simulink model "FirstDeb"  (R2022a)
settings: Solver=VariableStepAuto  StartTime=0.0  StopTime=Time*20000  RelTol=1e-3
InitFcn:
  | Time = 40;
values from neighbouring files (symbols this model uses):
  alpha = 0.4    [First.m]
  Fixeda = fi(a,1,13,12)    [First.m]
  FixedR = fi(R,1,8,6)    [First.m]
libraries: sim_stud_lib_r2022a x5, dspsrcs4 x2, dspsigops x2
settings Model: Creator=RolePups  LastModifiedBy=RolePups

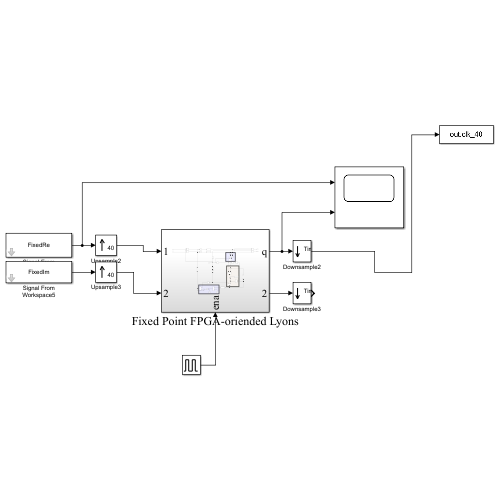
[thumbnail: Simulink's stored preview of the top-level diagram]
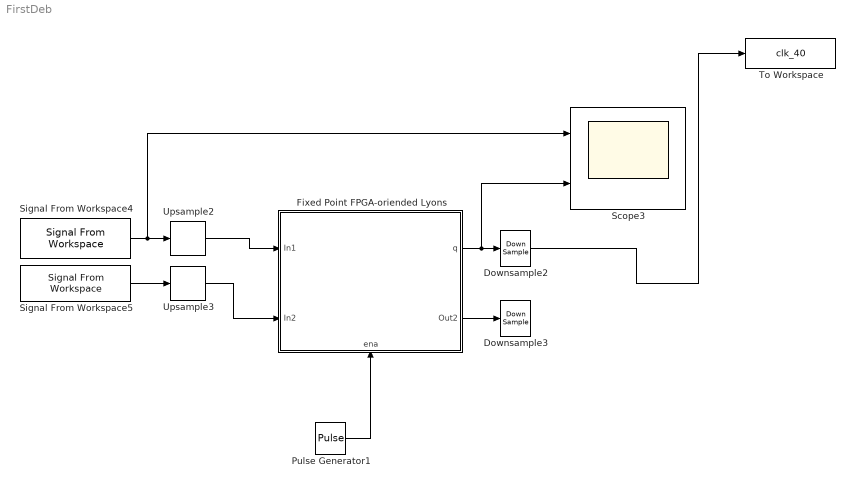
== system FirstDeb ==
  Downsample2 : DownSample  N=Time  RateOptions=Allow multirate processing
  Downsample3 : DownSample  N=Time  RateOptions=Allow multirate processing
  Fixed Point FPGA-oriended Lyons : Subsystem
      settings: PortSchema="{\"entries\":[{\"content\":{\"sides\":[{\"content\":{\"connectorIds\":[\"In1\",\"In2\"]},\"type\":\"ConnectorPlacement.EquallySpacedRectSide\",\"uuid\":\"2382ef4f-8b23-4fd9-9999-ae4ff3838c30\"},{\"content\":{\"connectorIds\":[\"Out1\",\"Out2\"],\"side\":\"RIGHT\"},\"type\":\"ConnectorPlacement.EquallySpacedRectSide\",\"uuid\":\"ff744322-ad90-46d9-948c-0637f52c7b9c\"},{\"content\":{\"connectorIds\":[],\"side\":\"TOP\"},\"type\":\"ConnectorPlacement.EquallySpacedRectSide\",\"uuid\":\"b0276f26-9e78-4e39-abf6-7a1348b88309\"},{\"content\":{\"connectorIds\":[\"In3\"],\"side\":\"BOTTOM\"},\"type\":\"ConnectorPlacement.EquallySpacedRectSide\",\"uuid\":\"b0dd70ff-8907-4b14-a46e-e3bbf4bdcae4\"}]},\"type\":\"ConnectorPlacement.EquallySpacedConnector\",\"uuid\":\"3f5cde89-4d4f-4bf7-b554-70cc79020603\"}],\"packageUris\":[\"http://schema.mathworks.com/mf0/Connector/R2020b\"],\"version\":\"1.0\"}"
  Pulse Generator1 : DiscretePulseGenerator  PulseType=Time based  Period=Time  PulseWidth=1/Time*100
  Scope3 : Scope  NumInputPorts=2
  Signal From Workspace4 : dspsrcs4/Signal From Workspace  X=FixedRe  Ts=Time  nsamps=1  OutputAfterFinalValue=Setting to zero  ignoreOrWarnInputAndFrameLengths=off  OutputFrames=off
  Signal From Workspace5 : dspsrcs4/Signal From Workspace  X=FixedIm  Ts=Time  nsamps=1  OutputAfterFinalValue=Setting to zero  ignoreOrWarnInputAndFrameLengths=off  OutputFrames=off
  To Workspace : ToWorkspace  VariableName=clk_40  SampleTime=-1
  Upsample2 : dspsigops/Upsample  N=Time  phase=0  RateOptions=Allow multirate processing  ic=0  mode=Unused parameter value
  Upsample3 : dspsigops/Upsample  N=Time  phase=0  RateOptions=Allow multirate processing  ic=0  mode=Unused parameter value
  wires:
  Fixed Point FPGA-oriended Lyons/1(q) -> Scope3/2, Downsample2/1
  Signal From Workspace5/1 -> Upsample3/1
  Upsample2/1 -> Fixed Point FPGA-oriended Lyons/1(In1)
  Fixed Point FPGA-oriended Lyons/2(Out2) -> Downsample3/1
  Pulse Generator1/1 -> Fixed Point FPGA-oriended Lyons/3(ena)
  Downsample2/1 -> To Workspace/1
  Signal From Workspace4/1 -> Scope3/1, Upsample2/1
  Upsample3/1 -> Fixed Point FPGA-oriended Lyons/2(In2)

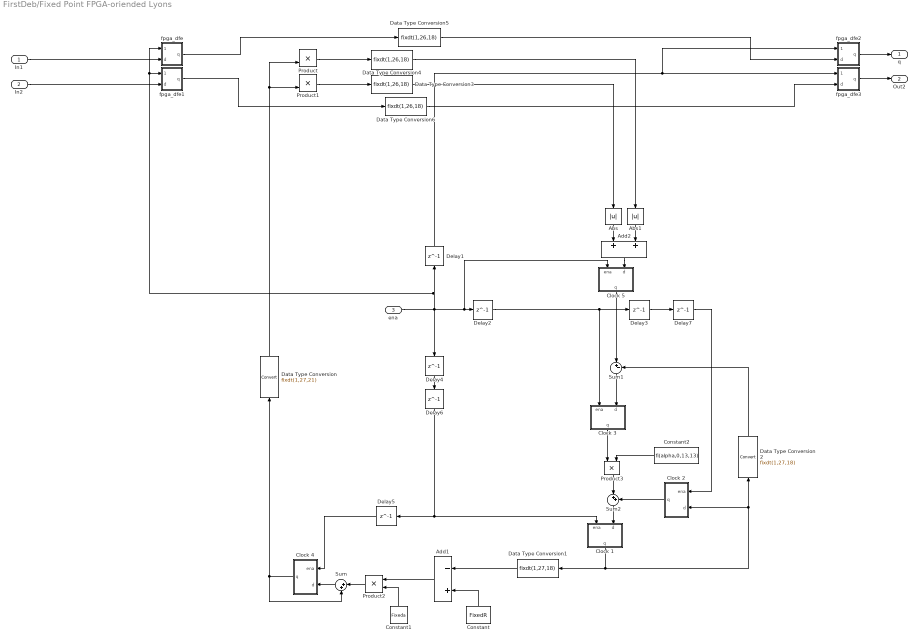
== system FirstDeb/Fixed Point FPGA-oriended Lyons ==
  In1 : Inport
  In2 : Inport  Port=2
  ena : Inport  Port=3
  Abs : Abs  OutDataTypeStr=fixdt(0,26,18)  SaturateOnIntegerOverflow=off
  Abs1 : Abs  OutDataTypeStr=fixdt(0,26,18)  SaturateOnIntegerOverflow=off
  Add1 : Sum  Inputs=-+  AccumDataTypeStr=fixdt(1,27,18)  OutDataTypeStr=fixdt(1,27,18)
  Add2 : Sum  AccumDataTypeStr=fixdt(0,27,18)  OutDataTypeStr=fixdt(0,27,18)
  Clock 1 : Subsystem
  Clock 2 : Subsystem
  Clock 3 : Subsystem
  Clock 4 : Subsystem
  Clock 5 : Subsystem
  Constant : Constant  Value=FixedR  SampleTime=-1
  Constant1 : Constant  Value=Fixeda  SampleTime=-1
  Constant2 : Constant  Value=fi(alpha,0,13,13)  SampleTime=-1
  Data Type Conversion : DataTypeConversion  OutDataTypeStr=fixdt(1,27,21)  SaturateOnIntegerOverflow=off  RndMeth=Floor
  Data Type Conversion1 : DataTypeConversion  OutDataTypeStr=fixdt(1,27,18)  SaturateOnIntegerOverflow=off  RndMeth=Floor
  Data Type Conversion2 : DataTypeConversion  OutDataTypeStr=fixdt(1,27,18)  SaturateOnIntegerOverflow=off  RndMeth=Floor
  Data Type Conversion{3..6} (4 alike) : DataTypeConversion  OutDataTypeStr=fixdt(1,26,18)  SaturateOnIntegerOverflow=off  RndMeth=Floor
  Delay{1..7} (7 alike) : Delay  DelayLength=1  InitialCondition=0
  Product : Product  OutDataTypeStr=fixdt(1,43,35)  LockScale=on
  Product1 : Product  OutDataTypeStr=fixdt(1,43,35)  LockScale=on
  Product2 : Product  OutDataTypeStr=fixdt(1,48,32)
  Product3 : Product  OutDataTypeStr=fixdt(1,48,32)
  Sum : Sum  Inputs=|++  AccumDataTypeStr=fixdt(1,48,32)  OutDataTypeStr=fixdt(1,48,32)
  Sum1 : Sum  Inputs=|+-  AccumDataTypeStr=fixdt(1,27,18)  OutDataTypeStr=fixdt(1,27,18)
  Sum2 : Sum  Inputs=|++  AccumDataTypeStr=fixdt(1,48,32)  OutDataTypeStr=fixdt(1,48,32)
  fpga_dfe : Subsystem  AncestorBlock=sim_stud_lib_r2022a/fpga_dfe
      mask Display:
      | disp('D');
      | port_label('input',1,'e');
      | port_label('input',2,'d');
      | port_label('output',1,'q');
  fpga_dfe1 : Subsystem  AncestorBlock=sim_stud_lib_r2022a/fpga_dfe
      mask Display:
      | disp('D');
      | port_label('input',1,'e');
      | port_label('input',2,'d');
      | port_label('output',1,'q');
  fpga_dfe2 : Subsystem  AncestorBlock=sim_stud_lib_r2022a/fpga_dfe
      mask Display:
      | disp('D');
      | port_label('input',1,'e');
      | port_label('input',2,'d');
      | port_label('output',1,'q');
  fpga_dfe3 : Subsystem  AncestorBlock=sim_stud_lib_r2022a/fpga_dfe
      mask Display:
      | disp('D');
      | port_label('input',1,'e');
      | port_label('input',2,'d');
      | port_label('output',1,'q');
  q : Outport
  Out2 : Outport  Port=2
  wires:
  Clock 4/1(q) -> Sum/2, Data Type Conversion/1
  Product/1 -> Data Type Conversion4/1
  Product1/1 -> Data Type Conversion3/1
  Constant/1 -> Add1/2
  Sum/1 -> Clock 4/2(d)
  Product2/1 -> Sum/1
  Constant1/1 -> Product2/2
  Abs1/1 -> Add2/2
  Abs/1 -> Add2/1
  Sum1/1 -> Clock 3/2(d)
  Constant2/1 -> Product3/2
  Product3/1 -> Sum2/1
  Clock 2/1(q) -> Sum2/2
  Add1/1 -> Product2/1
  Sum2/1 -> Clock 1/2(d)
  Clock 1/1(q) -> Data Type Conversion2/1, Clock 2/2(d), Data Type Conversion1/1
  Clock 3/1(q) -> Product3/1
  fpga_dfe2/1(q) -> q/1
  fpga_dfe3/1(q) -> Out2/1
  ena/1 -> Delay4/1, Delay1/1, fpga_dfe1/1(ena), fpga_dfe/1(ena), Clock 5/1(ena), Delay2/1
  Delay2/1 -> Delay3/1, Clock 3/1(ena)
  Delay3/1 -> Delay7/1
  Delay4/1 -> Delay6/1
  Delay5/1 -> Clock 4/1(ena)
  Delay7/1 -> Clock 2/1(ena)
  Add2/1 -> Clock 5/2(d)
  Clock 5/1(q) -> Sum1/1
  In1/1 -> fpga_dfe/2(d)
  In2/1 -> fpga_dfe1/2(d)
  Delay6/1 -> Clock 1/1(ena), Delay5/1
  Delay1/1 -> fpga_dfe3/1(ena), fpga_dfe2/1(ena)
  Data Type Conversion/1 -> Product/2, Product1/2
  Data Type Conversion1/1 -> Add1/1
  Data Type Conversion2/1 -> Sum1/2
  Data Type Conversion4/1 -> Abs1/1
  Data Type Conversion3/1 -> Abs/1
  fpga_dfe/1(q) -> Data Type Conversion5/1
  fpga_dfe1/1(q) -> Data Type Conversion6/1
  Data Type Conversion5/1 -> fpga_dfe2/2(d)
  Data Type Conversion6/1 -> fpga_dfe3/2(d)

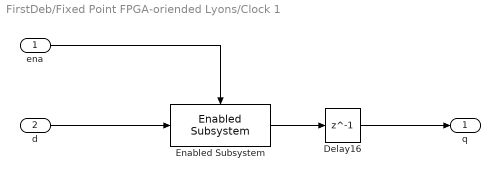
== system FirstDeb/Fixed Point FPGA-oriended Lyons/Clock 1 ==
  ena : Inport
  d : Inport  Port=2
  Delay16 : Delay  DelayLength=1
  Enabled Subsystem : sim_stud_lib_r2022a/fpga_dfe/Enabled Subsystem  SystemSampleTime=-1  VariantActivationTime=update diagram  Latency=0  AutoFrameSizeCalculation=off
  q : Outport  VectorParamsAs1DForOutWhenUnconnected=off
  wires:
  Delay16/1 -> q/1
  d/1 -> Enabled Subsystem/1
  Enabled Subsystem/1 -> Delay16/1
  ena/1 -> Enabled Subsystem/Enable

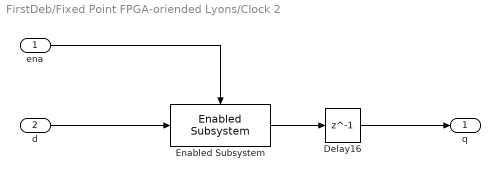
== system FirstDeb/Fixed Point FPGA-oriended Lyons/Clock 2 ==
  ena : Inport
  d : Inport  Port=2
  Delay16 : Delay  DelayLength=1
  Enabled Subsystem : sim_stud_lib_r2022a/fpga_dfe/Enabled Subsystem  SystemSampleTime=-1  VariantActivationTime=update diagram  Latency=0  AutoFrameSizeCalculation=off
  q : Outport  VectorParamsAs1DForOutWhenUnconnected=off
  wires:
  Delay16/1 -> q/1
  d/1 -> Enabled Subsystem/1
  Enabled Subsystem/1 -> Delay16/1
  ena/1 -> Enabled Subsystem/Enable

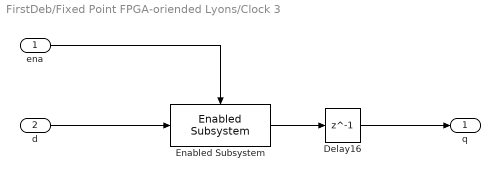
== system FirstDeb/Fixed Point FPGA-oriended Lyons/Clock 3 ==
  ena : Inport
  d : Inport  Port=2
  Delay16 : Delay  DelayLength=1
  Enabled Subsystem : sim_stud_lib_r2022a/fpga_dfe/Enabled Subsystem  SystemSampleTime=-1  VariantActivationTime=update diagram  Latency=0  AutoFrameSizeCalculation=off
  q : Outport  VectorParamsAs1DForOutWhenUnconnected=off
  wires:
  Delay16/1 -> q/1
  d/1 -> Enabled Subsystem/1
  Enabled Subsystem/1 -> Delay16/1
  ena/1 -> Enabled Subsystem/Enable

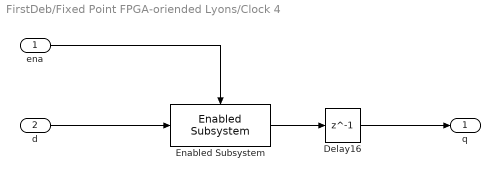
== system FirstDeb/Fixed Point FPGA-oriended Lyons/Clock 4 ==
  ena : Inport
  d : Inport  Port=2
  Delay16 : Delay  DelayLength=1
  Enabled Subsystem : sim_stud_lib_r2022a/fpga_dfe/Enabled Subsystem  SystemSampleTime=-1  VariantActivationTime=update diagram  Latency=0  AutoFrameSizeCalculation=off
  q : Outport  VectorParamsAs1DForOutWhenUnconnected=off
  wires:
  Delay16/1 -> q/1
  d/1 -> Enabled Subsystem/1
  Enabled Subsystem/1 -> Delay16/1
  ena/1 -> Enabled Subsystem/Enable

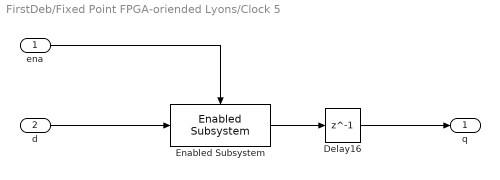
== system FirstDeb/Fixed Point FPGA-oriended Lyons/Clock 5 ==
  ena : Inport
  d : Inport  Port=2
  Delay16 : Delay  DelayLength=1
  Enabled Subsystem : sim_stud_lib_r2022a/fpga_dfe/Enabled Subsystem  SystemSampleTime=-1  VariantActivationTime=update diagram  Latency=0  AutoFrameSizeCalculation=off
  q : Outport  VectorParamsAs1DForOutWhenUnconnected=off
  wires:
  Delay16/1 -> q/1
  d/1 -> Enabled Subsystem/1
  Enabled Subsystem/1 -> Delay16/1
  ena/1 -> Enabled Subsystem/Enable

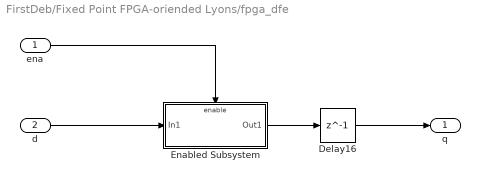
== system FirstDeb/Fixed Point FPGA-oriended Lyons/fpga_dfe ==
  ena : Inport
  d : Inport  Port=2
  Delay16 : Delay  DelayLength=1
  Enabled Subsystem : Subsystem  TreatAsAtomicUnit=on
  q : Outport  VectorParamsAs1DForOutWhenUnconnected=off
  wires:
  Enabled Subsystem/1(Out1) -> Delay16/1
  Delay16/1 -> q/1
  ena/1 -> Enabled Subsystem/Enable
  d/1 -> Enabled Subsystem/1(In1)

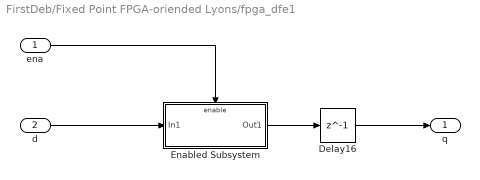
== system FirstDeb/Fixed Point FPGA-oriended Lyons/fpga_dfe1 ==
  ena : Inport
  d : Inport  Port=2
  Delay16 : Delay  DelayLength=1
  Enabled Subsystem : Subsystem  TreatAsAtomicUnit=on
  q : Outport  VectorParamsAs1DForOutWhenUnconnected=off
  wires:
  Enabled Subsystem/1(Out1) -> Delay16/1
  Delay16/1 -> q/1
  ena/1 -> Enabled Subsystem/Enable
  d/1 -> Enabled Subsystem/1(In1)

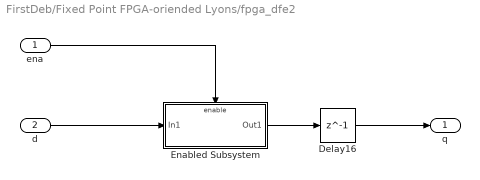
== system FirstDeb/Fixed Point FPGA-oriended Lyons/fpga_dfe2 ==
  ena : Inport
  d : Inport  Port=2
  Delay16 : Delay  DelayLength=1
  Enabled Subsystem : Subsystem  TreatAsAtomicUnit=on
  q : Outport  VectorParamsAs1DForOutWhenUnconnected=off
  wires:
  Enabled Subsystem/1(Out1) -> Delay16/1
  Delay16/1 -> q/1
  ena/1 -> Enabled Subsystem/Enable
  d/1 -> Enabled Subsystem/1(In1)

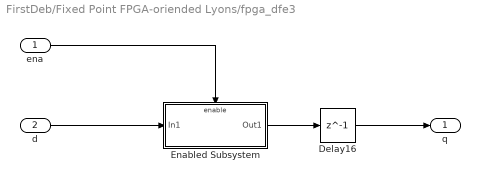
== system FirstDeb/Fixed Point FPGA-oriended Lyons/fpga_dfe3 ==
  ena : Inport
  d : Inport  Port=2
  Delay16 : Delay  DelayLength=1
  Enabled Subsystem : Subsystem  TreatAsAtomicUnit=on
  q : Outport  VectorParamsAs1DForOutWhenUnconnected=off
  wires:
  Enabled Subsystem/1(Out1) -> Delay16/1
  Delay16/1 -> q/1
  ena/1 -> Enabled Subsystem/Enable
  d/1 -> Enabled Subsystem/1(In1)

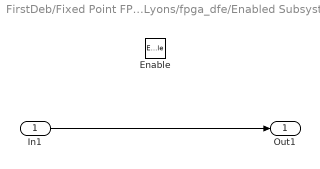
== system FirstDeb/Fixed Point FPGA-oriended Lyons/fpga_dfe/Enabled Subsystem ==
  In1 : Inport
  Enable : EnablePort
  Out1 : Outport  VectorParamsAs1DForOutWhenUnconnected=off
  wires:
  In1/1 -> Out1/1

== system FirstDeb/Fixed Point FPGA-oriended Lyons/fpga_dfe1/Enabled Subsystem ==
  In1 : Inport
  Enable : EnablePort
  Out1 : Outport  VectorParamsAs1DForOutWhenUnconnected=off
  wires:
  In1/1 -> Out1/1

== system FirstDeb/Fixed Point FPGA-oriended Lyons/fpga_dfe2/Enabled Subsystem ==
  In1 : Inport
  Enable : EnablePort
  Out1 : Outport  VectorParamsAs1DForOutWhenUnconnected=off
  wires:
  In1/1 -> Out1/1

== system FirstDeb/Fixed Point FPGA-oriended Lyons/fpga_dfe3/Enabled Subsystem ==
  In1 : Inport
  Enable : EnablePort
  Out1 : Outport  VectorParamsAs1DForOutWhenUnconnected=off
  wires:
  In1/1 -> Out1/1
